simulink model "Module7_NonlinearModel"  (R2016b)
settings: Solver=ode4  StartTime=0.0  StopTime=5000  FixedStep=0.1  RelTol=1e-3  EnableMultiTasking=on
undefined symbols (not defined in the file or in its folder): A1, A2, A3, c0, c1, c2, k, simSwitch, x0
settings Model: ExtModeTrigMode=oneshot  ExtModeArmWhenConnect=off  Creator=OJ  LastModifiedBy=HBM
settings DataIOCC: SaveFormat=Array  SignalLoggingSaveFormat=ModelDataLogs  StateSaveName=x  TimeSaveName=t  OutputSaveName=y
settings OptimizationCC: BooleanDataType=off  ExpressionDepthLimit=2147483647  InitFltsAndDblsToZero=on  LifeSpan=inf
settings DebuggingCC: SaveWithParameterizedLinksMsg=none  UnderspecifiedInitializationDetection=Classic  MergeDetectMultiDrivingBlocksExec=none  SignalResolutionControl=TryResolveAllWithWarning  MultiTaskCondExecSysMsg=none  FcnCallInpInsideContextMsg=warning  UnconnectedInputMsg=none  UnconnectedOutputMsg=none  UnconnectedLineMsg=none  StateNameClashWarn=warning  SFUnexpectedBacktrackingDiag=warning  SFNoUnconditionalDefaultTransitionDiag=warning  SFExecutionAtInitializationDiag=none
settings HardwareCC: ProdBitPerPointer=32  ProdBitPerSizeT=32  ProdBitPerPtrDiffT=32  ProdLargestAtomicFloat=None  ProdIntDivRoundTo=Undefined  ProdEndianess=Unspecified  ProdWordSize=32  ProdHWDeviceType=32-bit Generic  TargetUnknown=on
settings ModelReferenceCC: PropagateSignalLabelsOutOfModel=off
settings GRTTargetCC: TargetFcnLib=ansi_tfl_tmw.mat  TargetLangStandard=C89/C90 (ANSI)  GeneratePreprocessorConditionals=Disable all  CombineOutputUpdateFcns=off  GRTInterface=on
settings ConfigComp: CovMetricSettings=dw  CovHtmlReporting=on  CovSaveCumulativeToWorkspaceVar=on  CovSaveSingleToWorkspaceVar=on  CovExternalEMLEnable=off

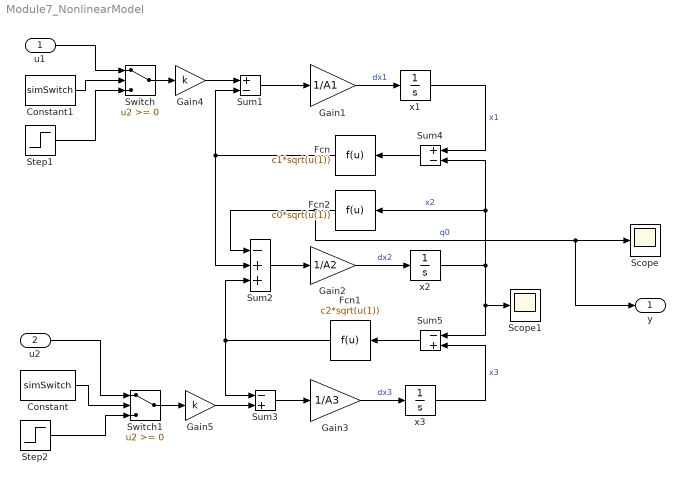
== system Module7_NonlinearModel ==
  u1 : Inport
  u2 : Inport  Port=2
  Constant : Constant  Value=simSwitch
  Constant1 : Constant  Value=simSwitch
  Fcn : Fcn  Expr=c1*sqrt(u(1))
  Fcn1 : Fcn  Expr=c2*sqrt(u(1))
  Fcn2 : Fcn  Expr=c0*sqrt(u(1))
  Gain1 : Gain  Gain=1/A1  SaturateOnIntegerOverflow=on  OutDataTypeStr=Inherit: Same as input  ParamDataTypeStr=Inherit: Same as input
  Gain2 : Gain  Gain=1/A2  SaturateOnIntegerOverflow=on  OutDataTypeStr=Inherit: Same as input  ParamDataTypeStr=Inherit: Same as input
  Gain3 : Gain  Gain=1/A3  SaturateOnIntegerOverflow=on  OutDataTypeStr=Inherit: Same as input  ParamDataTypeStr=Inherit: Same as input
  Gain4 : Gain  Gain=k  SaturateOnIntegerOverflow=on  OutDataTypeStr=Inherit: Same as input  ParamDataTypeStr=Inherit: Same as input
  Gain5 : Gain  Gain=k  SaturateOnIntegerOverflow=on  OutDataTypeStr=Inherit: Same as input  ParamDataTypeStr=Inherit: Same as input
  Scope : Scope
  Scope1 : Scope
  Step1 : Step  Time=0  Before=u  After=u  SampleTime=0.1
  Step2 : Step  Time=0  Before=u  After=u  SampleTime=0.1
  Sum1 : Sum  Inputs=+-  SaturateOnIntegerOverflow=on  InputSameDT=on  OutDataTypeStr=Inherit: Same as first input
  Sum2 : Sum  Inputs=-++  SaturateOnIntegerOverflow=on  InputSameDT=on  OutDataTypeStr=Inherit: Same as first input
  Sum3 : Sum  Inputs=-+  SaturateOnIntegerOverflow=on  InputSameDT=on  OutDataTypeStr=Inherit: Same as first input
  Sum4 : Sum  Inputs=+-  SaturateOnIntegerOverflow=on  InputSameDT=on  OutDataTypeStr=Inherit: Same as first input
  Sum5 : Sum  Inputs=-+  SaturateOnIntegerOverflow=on  InputSameDT=on  OutDataTypeStr=Inherit: Same as first input
  Switch : Switch  SaturateOnIntegerOverflow=on  InputSameDT=on
  Switch1 : Switch  SaturateOnIntegerOverflow=on  InputSameDT=on
  x1 : Integrator  Priority=1  InitialCondition=x0(1)
  x2 : Integrator  Priority=2  InitialCondition=x0(2)
  x3 : Integrator  Priority=3  InitialCondition=x0(3)
  y : Outport
  wires:
  Gain1/1 -> x1/1  "dx1"
  Gain2/1 -> x2/1  "dx2"
  Gain3/1 -> x3/1  "dx3"
  Sum1/1 -> Gain1/1
  Sum2/1 -> Gain2/1
  Sum3/1 -> Gain3/1
  x1/1 -> Sum4/1  "x1"
  x2/1 -> Sum4/2, Fcn2/1, Sum5/1, Scope1/1  "x2"
  x3/1 -> Sum5/2  "x3"
  Sum4/1 -> Fcn/1
  Sum5/1 -> Fcn1/1
  Fcn/1 -> Sum1/2, Sum2/2
  Fcn2/1 -> Scope/1, y/1, Sum2/1  "q0"
  Fcn1/1 -> Sum2/3, Sum3/1
  Gain4/1 -> Sum1/1
  Gain5/1 -> Sum3/2
  Switch/1 -> Gain4/1
  Step1/1 -> Switch/3
  Switch1/1 -> Gain5/1
  Step2/1 -> Switch1/3
  u1/1 -> Switch/1
  u2/1 -> Switch1/1
  Constant/1 -> Switch1/2
  Constant1/1 -> Switch/2
